simulink model "SMC"  (R2024b)
settings: Solver=FixedStepAuto  StartTime=0.0  StopTime=200  FixedStep=1e-3  RelTol=1e-3
undefined symbols (not defined in the file): Orientation, Position
libraries: robotlib x3, simulink_extras x3, sharedutil x2
(part 2 of 2)

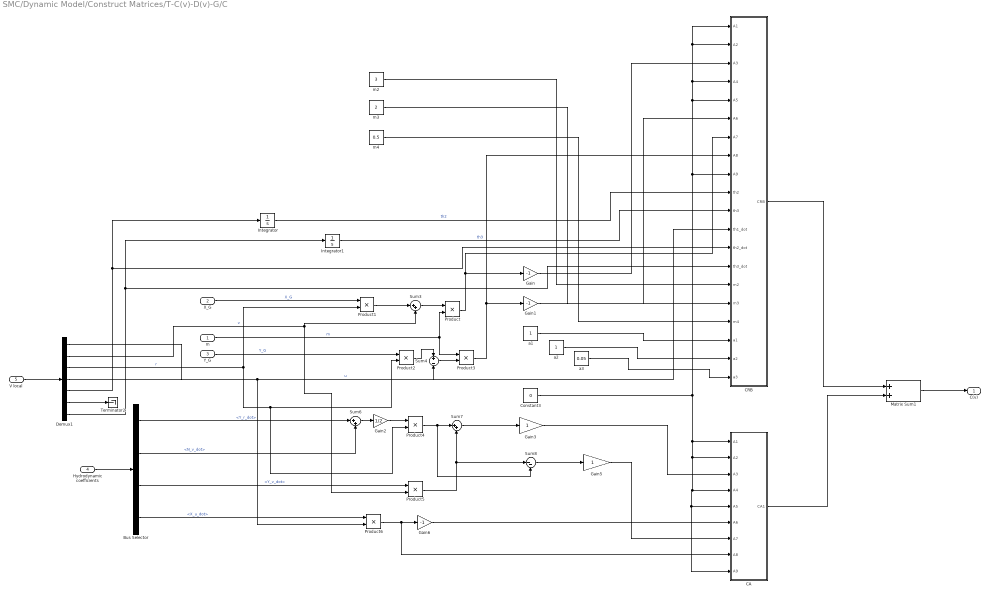
== system SMC/Dynamic Model/Construct Matrices/T-C(v)-D(v)-G/C ==
  m : Inport
  X_G : Inport  Port=2
  Y_G : Inport  Port=3
  Hydrodynamic coefficients : Inport  Port=4
  V local : Inport  Port=5
  Bus Selector : BusSelector  OutputSignals=Y_r_dot,N_v_dot,Y_v_dot,X_u_dot
  CA : MATLAB Function  TreatAsAtomicUnit=on
  CRB : MATLAB Function  TreatAsAtomicUnit=on
  Constant3 : Constant  Value=0
  Demux1 : Demux  Outputs=7
  Gain : Gain  Gain=-1
  Gain1 : Gain  Gain=-1
  Gain2 : Gain  Gain=1/2
  Gain3 : Gain
  Gain5 : Gain
  Gain6 : Gain  Gain=-1
  Integrator : Integrator
  Integrator1 : Integrator
  Matrix Sum1 : Sum
  Product{,1..6} (7 alike) : Product
  Sum3 : Sum  Inputs=|++
  Sum4 : Sum  Inputs=+-
  Sum6 : Sum  Inputs=|++
  Sum7 : Sum  Inputs=|++
  Sum8 : Sum  Inputs=|--
  Terminator2 : Terminator
  a1 : Constant
  a2 : Constant
  a3 : Constant  Value=0.05
  m2 : Constant  Value=3
  m3 : Constant  Value=2
  m4 : Constant  Value=0.5
  C(v) : Outport
  wires:
  Hydrodynamic coefficients/1 -> Bus Selector/1
  Demux1/1 -> Product6/2, Sum4/2  "u"
  Gain3/1 -> CA/3(A3)
  CRB/1(CRB) -> Matrix Sum1/1
  Demux1/4 -> CRB/12(th1_dot)
  Product1/1 -> Sum3/1
  Gain6/1 -> CA/6(A6)
  Constant3/1 -> CRB/9(A9), CRB/2(A2), CRB/1(A1), CRB/4(A4), CRB/5(A5), CA/4(A4), CA/5(A5), CA/9(A9), CA/2(A2), CA/1(A1)
  Bus Selector/1 -> Sum6/1  "<Y_r_dot>"
  Product6/1 -> Gain6/1, CA/8(A8)
  Y_G/1 -> Product2/1  "Y_G"
  Sum3/1 -> Product/1
  Demux1/2 -> Product5/2, Sum3/2  "v"
  Bus Selector/2 -> Sum6/2  "<N_v_dot>"
  Demux1/7 -> Integrator1/1, CRB/14(th3_dot)
  Gain1/1 -> CRB/6(A6)
  Sum6/1 -> Gain2/1
  X_G/1 -> Product1/1  "X_G"
  Product5/1 -> Sum7/2, Sum8/1
  Demux1/6 -> Terminator2/1
  Gain2/1 -> Product4/1
  Bus Selector/4 -> Product6/1  "<X_u_dot>"
  Product3/1 -> Gain1/1, CRB/8(A8)
  m/1 -> Product/2, Product3/1  "m"
  Gain/1 -> CRB/3(A3)
  Demux1/5 -> CRB/13(th2_dot), Integrator/1
  Product/1 -> Gain/1, CRB/7(A7)
  Product2/1 -> Sum4/1
  Demux1/3 -> Product1/2, Product2/2, Product4/2  "r"
  Sum7/1 -> Gain3/1
  Sum8/1 -> Gain5/1
  Bus Selector/3 -> Product5/1  "<Y_v_dot>"
  CA/1(CA1) -> Matrix Sum1/2
  Matrix Sum1/1 -> C(v)/1
  Gain5/1 -> CA/7(A7)
  Sum4/1 -> Product3/2
  V local/1 -> Demux1/1
  Product4/1 -> Sum7/1, Sum8/2
  Integrator/1 -> CRB/10(th2)  "th2"
  Integrator1/1 -> CRB/11(th3)  "th3"
  m2/1 -> CRB/15(m2)
  m3/1 -> CRB/16(m3)
  m4/1 -> CRB/17(m4)
  a1/1 -> CRB/18(a1)
  a2/1 -> CRB/19(a2)
  a3/1 -> CRB/20(a3)

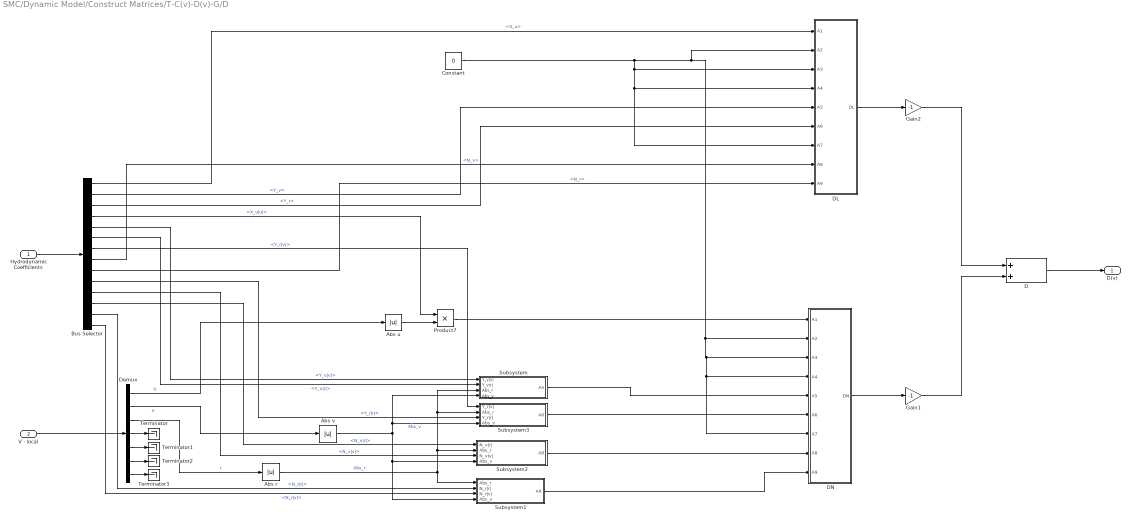
== system SMC/Dynamic Model/Construct Matrices/T-C(v)-D(v)-G/D ==
  note: u
  note: v
  Hydrodynamic Coefficients : Inport
  V - local : Inport  Port=2
  Abs r : Abs  SaturateOnIntegerOverflow=off
  Abs u : Abs  SaturateOnIntegerOverflow=off
  Abs v : Abs  SaturateOnIntegerOverflow=off
  Bus Selector : BusSelector  OutputSignals=X_u,Y_v,Y_r,X_u|u|,Y_v|v|,Y_v|r|,Y_r|v|,N_v,N_r,Y_r|r|,N_v|v|,N_v|r|,N_r|r|,N_r|v|
  Constant : Constant  Value=0
  D : Sum
  DL : MATLAB Function  TreatAsAtomicUnit=on
  DN : MATLAB Function  TreatAsAtomicUnit=on
  Demux : Demux  Outputs=7
  Gain1 : Gain  Gain=-1
  Gain2 : Gain  Gain=-1
  Product7 : Product
  Subsystem : Subsystem
  Subsystem1 : Subsystem
  Subsystem2 : Subsystem
  Subsystem3 : Subsystem
  Terminator{,1..3} (4 alike) : Terminator
  D(v) : Outport
  wires:
  Demux/7 -> Terminator3/1
  Hydrodynamic Coefficients/1 -> Bus Selector/1
  Demux/6 -> Terminator2/1
  Demux/5 -> Terminator1/1
  Demux/1 -> Abs u/1
  Demux/4 -> Terminator/1
  Bus Selector/5 -> Subsystem/1("Y_v|v| ")  "<Y_v|v|>"
  Demux/2 -> Abs v/1
  Abs r/1 -> Subsystem/3(Abs_r), Subsystem3/2("Abs_r "), Subsystem2/2(Abs_r), Subsystem1/1(Abs_r)  "Abs_r"
  Gain1/1 -> D/2
  DL/1(DL) -> Gain2/1
  DN/1(DN) -> Gain1/1
  V - local/1 -> Demux/1
  Bus Selector/6 -> Subsystem/2(Y_v|r|)  "<Y_v|r|>"
  Demux/3 -> Abs r/1  "r"
  D/1 -> D(v)/1
  Gain2/1 -> D/1
  Subsystem2/1(A8) -> DN/8(A8)
  Bus Selector/4 -> Product7/1  "<X_u|u|>"
  Bus Selector/13 -> Subsystem1/2(N_r|r|)  "<N_r|r|>"
  Bus Selector/11 -> Subsystem2/3(N_v|v|)  "<N_v|v|>"
  Bus Selector/12 -> Subsystem2/1(N_v|r|)  "<N_v|r|>"
  Subsystem1/1(A9) -> DN/9(A9)
  Bus Selector/7 -> Subsystem3/1(Y_r|v|)  "<Y_r|v|>"
  Abs v/1 -> Subsystem/4("Abs_v "), Subsystem3/4(Abs_v), Subsystem1/4(Abs_v), Subsystem2/4(Abs_v)  "Abs_v"
  Constant/1 -> DL/2(A2), DN/2(A2), DN/3(A3), DN/4(A4), DN/7(A7), DL/4(A4), DL/7(A7), DL/3(A3)
  Bus Selector/14 -> Subsystem1/3(N_r|v|)  "<N_r|v|>"
  Abs u/1 -> Product7/2
  Subsystem/1(A5) -> DN/5(A5)
  Bus Selector/1 -> DL/1(A1)  "<X_u>"
  Subsystem3/1(A6) -> DN/6(A6)
  Product7/1 -> DN/1(A1)
  Bus Selector/10 -> Subsystem3/3(Y_r|r|)  "<Y_r|r|>"
  Bus Selector/9 -> DL/9(A9)  "<N_r>"
  Bus Selector/8 -> DL/8(A8)  "<N_v>"
  Bus Selector/3 -> DL/6(A6)  "<Y_r>"
  Bus Selector/2 -> DL/5(A5)  "<Y_v>"

== system SMC/Dynamic Model/Construct Matrices/T-C(v)-D(v)-G/Tau ==
  B : Inport
  Tport : Inport  Port=2
  Tstbd : Inport  Port=3
  q1 : Inport  Port=4
  q2 : Inport  Port=5
  q3 : Inport  Port=6
  q4 : Inport  Port=7
  Mux : Mux  Inputs=7
  Product25 : Product
  Sum : Sum  Inputs=|++
  Sum1 : Sum  Inputs=|+-
  Ty : Constant  Value=0
  Tz : Gain  Gain=1/2
  T : Outport  VectorParamsAs1DForOutWhenUnconnected=off
  wires:
  Tstbd/1 -> Sum/2, Sum1/2  "Tstbd"
  q3/1 -> Mux/6
  q2/1 -> Mux/5
  q1/1 -> Mux/4
  Tz/1 -> Mux/3  "Tz"
  Product25/1 -> Tz/1
  Sum1/1 -> Product25/2
  Mux/1 -> T/1  "T"
  Tport/1 -> Sum/1, Sum1/1  "Tport"
  Ty/1 -> Mux/2  "Ty"
  Sum/1 -> Mux/1
  q4/1 -> Mux/7
  B/1 -> Product25/1  "B"

== system SMC/Controller/Construct Matrices/C(v)D(v)G/D/Subsystem ==
  "Y_v|v| " : Inport
  Y_v|r| : Inport  Port=2
  Abs_r : Inport  Port=3
  "Abs_v " : Inport  Port=4
  Product8 : Product
  Product9 : Product
  Sum10 : Sum  Inputs=|++
  A5 : Outport  VectorParamsAs1DForOutWhenUnconnected=off
  wires:
  Y_v|r|/1 -> Product9/1
  Abs_r/1 -> Product9/2
  Product9/1 -> Sum10/2
  "Y_v|v| "/1 -> Product8/1
  Product8/1 -> Sum10/1
  "Abs_v "/1 -> Product8/2
  Sum10/1 -> A5/1

== system SMC/Controller/Construct Matrices/C(v)D(v)G/D/Subsystem1 ==
  Abs_r : Inport
  N_r|r| : Inport  Port=2
  N_r|v| : Inport  Port=3
  Abs_v : Inport  Port=4
  Product14 : Product
  Product15 : Product
  Sum13 : Sum  Inputs=|++
  A9 : Outport  VectorParamsAs1DForOutWhenUnconnected=off
  wires:
  Product15/1 -> Sum13/1
  Sum13/1 -> A9/1
  N_r|v|/1 -> Product14/1
  Product14/1 -> Sum13/2
  Abs_r/1 -> Product15/2
  N_r|r|/1 -> Product15/1
  Abs_v/1 -> Product14/2

== system SMC/Controller/Construct Matrices/C(v)D(v)G/D/Subsystem2 ==
  N_v|r| : Inport
  Abs_r : Inport  Port=2
  N_v|v| : Inport  Port=3
  Abs_v : Inport  Port=4
  Product12 : Product
  Product13 : Product
  Sum12 : Sum  Inputs=|++
  A8 : Outport  VectorParamsAs1DForOutWhenUnconnected=off
  wires:
  Sum12/1 -> A8/1
  Product13/1 -> Sum12/1
  N_v|v|/1 -> Product12/1
  Product12/1 -> Sum12/2
  Abs_r/1 -> Product13/2
  Abs_v/1 -> Product12/2
  N_v|r|/1 -> Product13/1

== system SMC/Controller/Construct Matrices/C(v)D(v)G/D/Subsystem3 ==
  Y_r|v| : Inport
  "Abs_r " : Inport  Port=2
  Y_r|r| : Inport  Port=3
  Abs_v : Inport  Port=4
  Product10 : Product
  Product11 : Product
  Sum11 : Sum  Inputs=|++
  A6 : Outport  VectorParamsAs1DForOutWhenUnconnected=off
  wires:
  Product11/1 -> Sum11/2
  Product10/1 -> Sum11/1
  Sum11/1 -> A6/1
  Y_r|v|/1 -> Product10/1
  "Abs_r "/1 -> Product11/2
  Y_r|r|/1 -> Product11/1
  Abs_v/1 -> Product10/2

== system SMC/Dynamic Model/Construct Matrices/T-C(v)-D(v)-G/D/Subsystem ==
  "Y_v|v| " : Inport
  Y_v|r| : Inport  Port=2
  Abs_r : Inport  Port=3
  "Abs_v " : Inport  Port=4
  Product8 : Product
  Product9 : Product
  Sum10 : Sum  Inputs=|++
  A5 : Outport  VectorParamsAs1DForOutWhenUnconnected=off
  wires:
  Y_v|r|/1 -> Product9/1
  Abs_r/1 -> Product9/2
  Product9/1 -> Sum10/2
  "Y_v|v| "/1 -> Product8/1
  Product8/1 -> Sum10/1
  "Abs_v "/1 -> Product8/2
  Sum10/1 -> A5/1

== system SMC/Dynamic Model/Construct Matrices/T-C(v)-D(v)-G/D/Subsystem1 ==
  Abs_r : Inport
  N_r|r| : Inport  Port=2
  N_r|v| : Inport  Port=3
  Abs_v : Inport  Port=4
  Product14 : Product
  Product15 : Product
  Sum13 : Sum  Inputs=|++
  A9 : Outport  VectorParamsAs1DForOutWhenUnconnected=off
  wires:
  Product15/1 -> Sum13/1
  Sum13/1 -> A9/1
  N_r|v|/1 -> Product14/1
  Product14/1 -> Sum13/2
  Abs_r/1 -> Product15/2
  N_r|r|/1 -> Product15/1
  Abs_v/1 -> Product14/2

== system SMC/Dynamic Model/Construct Matrices/T-C(v)-D(v)-G/D/Subsystem2 ==
  N_v|r| : Inport
  Abs_r : Inport  Port=2
  N_v|v| : Inport  Port=3
  Abs_v : Inport  Port=4
  Product12 : Product
  Product13 : Product
  Sum12 : Sum  Inputs=|++
  A8 : Outport  VectorParamsAs1DForOutWhenUnconnected=off
  wires:
  Sum12/1 -> A8/1
  Product13/1 -> Sum12/1
  N_v|v|/1 -> Product12/1
  Product12/1 -> Sum12/2
  Abs_r/1 -> Product13/2
  Abs_v/1 -> Product12/2
  N_v|r|/1 -> Product13/1

== system SMC/Dynamic Model/Construct Matrices/T-C(v)-D(v)-G/D/Subsystem3 ==
  Y_r|v| : Inport
  "Abs_r " : Inport  Port=2
  Y_r|r| : Inport  Port=3
  Abs_v : Inport  Port=4
  Product10 : Product
  Product11 : Product
  Sum11 : Sum  Inputs=|++
  A6 : Outport  VectorParamsAs1DForOutWhenUnconnected=off
  wires:
  Product11/1 -> Sum11/2
  Product10/1 -> Sum11/1
  Sum11/1 -> A6/1
  Y_r|v|/1 -> Product10/1
  "Abs_r "/1 -> Product11/2
  Y_r|r|/1 -> Product11/1
  Abs_v/1 -> Product10/2

== matlab function SMC/MATLAB Function4 ==
  data: qw input; XYZ output; qx input; qy input; qz input
function XYZ = fcn(qw, qx, qy, qz)
quat = [qw qx qy qz];
XYZ = quat2eul(quat);

== matlab function SMC/Wave Disturbance ==
  data: t input; tau_wave output
function tau_wave = WaveDisturbance3DOF(t)
%#codegen
% Simulink-compatible wave disturbance force/torque for 3DOF USV

% Constants
rho = 1000;      % Water density [kg/m^3]
g = 9.81;        % Gravity [m/s^2]
L = 4.29;        % Length overall [m]
B = 2.20;        % Beam [m]
T = 0.105;       % Draft [m]
x_G = 1.27;      % CG longitudinal [m]

% Wave heading (0 = surge, pi/2 = sway)
beta = pi/4;     % 45 degrees in radians

% Wave properties (3 harmonic components)
A = [0.03, 0.04, 0.02];                % Amplitudes [m]
lambda = [2.0, 3.0, 1.5];             % Wavelengths [m]
omega = sqrt(g * 2 * pi ./ lambda);   % Angular frequencies [rad/s]
phi = [0, pi/4, pi/2];                % Phases

% Initialize slope s_i(t)
s = zeros(1,3);
for i = 1:3
    s(i) = (A(i)/(2*pi*lambda(i))) * sin(omega(i)*t + phi(i));
end

% Compute wave-induced forces
X_wave = sum(rho * g * B * L * T * cos(beta) * s);
Y_wave = -sum(rho * g * B * L * T * sin(beta) * s);
N_wave = sum((1/24) * rho * g * B * L * (L^2 - B^2) * sin(2*beta) * s.^2);

% Output vector
tau_wave = [X_wave; Y_wave; N_wave; 0; 0; 0; 0];

== matlab function SMC/Controller/Subsystem5/MATLAB Function ==
  data: A1 input; A2 input; A3 input; A4 input; A5 input; A6 input; A7 input; A8 input; A9 input; J1 output
function J1 = fcn(A1, A2, A3, A4, A5, A6, A7, A8, A9)

J1 = [A1,A2,A3,0,0,0,0;
    A4,A5,A6,0,0,0,0;
    A7,A8,A9,0,0,0,0;
    0,0,0,1,0,0,0;
    0,0,0,0,1,0,0;
    0,0,0,0,0,1,0;
    0,0,0,0,0,0,1;];

== matlab function SMC/Dynamic Model/Construct Matrices/M/MATLAB Function ==
  data: A1 input; A2 input; A3 input; A4 input; A5 input; A6 input; A7 input; A8 input; A9 input; M output; m1 input; m2 input; m3 input; m4 input; a1 input; a2 input; a3 input; th2 input; th3 input
function M = fcn(A1, A2, A3, A4, A5, A6, A7, A8, A9, m1, m2, m3, m4, a1, a2, a3, th2, th3)

% Define the expressions for M
m11 = (a1^2*m1)/4 + a1^2*m2 + a1^2*m3 + (a2^2*m2)/4 + a1^2*m4 + a2^2*m3 + a2^2*m4 + a3^2*m4 + 2*a1*a3*m4*cos(th2 + th3) + a1*a2*m2*cos(th2) + 2*a1*a2*m3*cos(th2) + 2*a1*a2*m4*cos(th2) + 2*a2*a3*m4*cos(th3);
m12 = (a2^2*m2)/4 + a2^2*m3 + a2^2*m4 + a3^2*m4 + a1*a3*m4*cos(th2 + th3) + (a1*a2*m2*cos(th2))/2 + a1*a2*m3*cos(th2) + a1*a2*m4*cos(th2) + 2*a2*a3*m4*cos(th3);
m13 = 0;
m14 = a3^2*m4 + a1*a3*m4*cos(th2 + th3) + a2*a3*m4*cos(th3);
m21 = (a2^2*m2)/4 + a2^2*m3 + a2^2*m4 + a3^2*m4 + a1*a3*m4*cos(th2 + th3) + (a1*a2*m2*cos(th2))/2 + a1*a2*m3*cos(th2) + a1*a2*m4*cos(th2) + 2*a2*a3*m4*cos(th3);
m22 = (a2^2*m2)/4 + a2^2*m3 + a2^2*m4 + a3^2*m4 + 2*a2*a3*m4*cos(th3);
m23 = 0;
m24 = m4*a3^2 + a2*m4*cos(th3)*a3;
m31 = 0;
m32 = 0;
m33 = (m3 + 4*m4)/4;
m34 = 0;
m41 = a3^2*m4 + a3*m4*a1*cos(th2 + th3) + a3*m4*a2*cos(th3);
m42 = a3^2*m4 + a3*m4*a2*cos(th3);
m43 = 0;
m44 = a3^2*m4;

M = [A1,A2,A3,0,0,0,0;
    A4,A5,A6,0,0,0,0;
    A7,A8,A9,0,0,0,0;
    0,0,0,m11,m12,m13,m14;
    0,0,0,m21,m22,m23,m24;
    0,0,0,m31,m32,m33,m34;
    0,0,0,m41,m42,m43,m44];

== matlab function SMC/Dynamic Model/Construct Matrices/M^-1 ==
  data: u input; y output
function y = fcn(u)
y = inv(u);

== matlab function SMC/Dynamic Model/Construct Matrices/T-C(v)-D(v)-G/C/CA ==
  data: A1 input; A2 input; A3 input; A4 input; A5 input; A6 input; A7 input; A8 input; A9 input; CA1 output
function CA1 = fcn(A1, A2, A3, A4, A5, A6, A7, A8, A9)

CA1 = [A1,A2,A3,0,0,0,0;
    A4,A5,A6,0,0,0,0;
    A7,A8,A9,0,0,0,0;
    0,0,0,0,0,0,0;
    0,0,0,0,0,0,0;
    0,0,0,0,0,0,0;
    0,0,0,0,0,0,0;];

== matlab function SMC/Dynamic Model/Construct Matrices/T-C(v)-D(v)-G/C/CRB ==
  data: A1 input; A2 input; A3 input; A4 input; A5 input; A6 input; A7 input; A8 input; A9 input; CRB output; th2 input; th3 input; th1_dot input; th2_dot input; th3_dot input; m2 input; m3 input; m4 input; a1 input; a2 input; a3 input
function CRB = fcn(A1, A2, A3, A4, A5, A6, A7, A8, A9, th2, th3, th1_dot, th2_dot, th3_dot, m2, m3, m4, a1, a2, a3)

% Define the expressions for C
c11 = -2*a1*a3*m4*sin(th2 + th3) + th2_dot + th3_dot - a1*a2*m2*sin(th2) - 2*a1*a2*m3*sin(th2) - 2*a1*a2*m4*sin(th2) - 2*a2*a3*m4*sin(th3);
c12 = -a1*a3*m4*sin(th2 + th3) + th2_dot + th3_dot - (a1*a2*m2*sin(th2))/2 - a1*a2*m3*sin(th2) - a1*a2*m4*sin(th2) - 2*a2*a3*m4*sin(th3);
c13 = 0;
c14 = -a1*a3*m4*sin(th2 + th3) + th2_dot + th3_dot - a2*a3*m4*sin(th3);
c21 = ((a1*(a2*m2*sin(th2) + 2*a2*m3*sin(th2) + 2*a2*m4*sin(th2) + 2*a3*m4*sin(th2 + th3)))/2)*th1_dot + - a1*a3*m4*sin(th2 + th3) - (a1*a2*m2*sin(th2))/2 - a1*a2*m3*sin(th2) - a1*a2*m4*sin(th2) - 2*a2*a3*m4*sin(th3);
c22 = ((a1*(a2*m2*sin(th2) + 2*a2*m3*sin(th2) + 2*a2*m4*sin(th2) + 2*a3*m4*sin(th2 + th3)))/2 + 1)*th1_dot - 2*a2*a3*m4*sin(th3);
c23 = 0;
c24 = (a1*a3*m4*sin(th2 + th3) + 1)*th1_dot - a2*a3*m4*sin(th3);
c31 = 0;
c32 = 0;
c33 = 0;
c34 = 0;
c41 = a2*sin(th3)*th1_dot - a1*a3*m4*sin(th2 + th3) - a2*a3*m4*sin(th3);
c42 = (a3*m4*(a1*sin(th2 + th3) + a2*sin(th3)) + a2*a3*m4*sin(th3) + 1)*th1_dot + a2*a3*m4*sin(th3)*th2_dot -a2*a3*m4*sin(th3);
c43 = 0;
c44 = a2*a3*m4*sin(th3)*th2_dot + (a3*m4*(a1*sin(th2 + th3) + a2*sin(th3)) + 1)*th1_dot;

CRB = [A1,A2,A3,0,0,0,0;
    A4,A5,A6,0,0,0,0;
    A7,A8,A9,0,0,0,0;
    0,0,0,c11,c12,c13,c14;
    0,0,0,c21,c22,c23,c24;
    0,0,0,c31,c32,c33,c34;
    0,0,0,c41,c42,c43,c44];

== matlab function SMC/Dynamic Model/Construct Matrices/T-C(v)-D(v)-G/D/DL ==
  data: A1 input; A2 input; A3 input; A4 input; A5 input; A6 input; A7 input; A8 input; A9 input; DL output
function DL = fcn(A1, A2, A3, A4, A5, A6, A7, A8, A9)

DL = [A1,A2,A3,0,0,0,0;
    A4,A5,A6,0,0,0,0;
    A7,A8,A9,0,0,0,0;
    0,0,0,0,0,0,0;
    0,0,0,0,0,0,0;
    0,0,0,0,0,0,0;
    0,0,0,0,0,0,0;];

== matlab function SMC/Dynamic Model/Construct Matrices/T-C(v)-D(v)-G/D/DN ==
  data: A1 input; A2 input; A3 input; A4 input; A5 input; A6 input; A7 input; A8 input; A9 input; DN output
function DN = fcn(A1, A2, A3, A4, A5, A6, A7, A8, A9)

DN = [A1,A2,A3,0,0,0,0;
    A4,A5,A6,0,0,0,0;
    A7,A8,A9,0,0,0,0;
    0,0,0,0,0,0,0;
    0,0,0,0,0,0,0;
    0,0,0,0,0,0,0;
    0,0,0,0,0,0,0];

== matlab function SMC/Dynamic Model/Construct Matrices/T-C(v)-D(v)-G/G ==
  data: m3 input; G output; m4 input; g input
function G = fcn(m3, m4, g)

% Define the expressions for G
g1 = 0
g2 = 0
g3 = g*(m3 + m4)
g4 = 0

G = [0;0;0;g1;g2;g3;g4];

== matlab function SMC/Controller/Construct Matrices/M2/MATLAB Function ==
  data: A1 input; A2 input; A3 input; A4 input; A5 input; A6 input; A7 input; A8 input; A9 input; M output; m1 input; m2 input; m3 input; m4 input; a1 input; a2 input; a3 input; th2 input; th3 input
function M = fcn(A1, A2, A3, A4, A5, A6, A7, A8, A9, m1, m2, m3, m4, a1, a2, a3, th2, th3)

% Define the expressions for M
m11 = (a1^2*m1)/4 + a1^2*m2 + a1^2*m3 + (a2^2*m2)/4 + a1^2*m4 + a2^2*m3 + a2^2*m4 + a3^2*m4 + 2*a1*a3*m4*cos(th2 + th3) + a1*a2*m2*cos(th2) + 2*a1*a2*m3*cos(th2) + 2*a1*a2*m4*cos(th2) + 2*a2*a3*m4*cos(th3);
m12 = (a2^2*m2)/4 + a2^2*m3 + a2^2*m4 + a3^2*m4 + a1*a3*m4*cos(th2 + th3) + (a1*a2*m2*cos(th2))/2 + a1*a2*m3*cos(th2) + a1*a2*m4*cos(th2) + 2*a2*a3*m4*cos(th3);
m13 = 0;
m14 = a3^2*m4 + a1*a3*m4*cos(th2 + th3) + a2*a3*m4*cos(th3);
m21 = (a2^2*m2)/4 + a2^2*m3 + a2^2*m4 + a3^2*m4 + a1*a3*m4*cos(th2 + th3) + (a1*a2*m2*cos(th2))/2 + a1*a2*m3*cos(th2) + a1*a2*m4*cos(th2) + 2*a2*a3*m4*cos(th3);
m22 = (a2^2*m2)/4 + a2^2*m3 + a2^2*m4 + a3^2*m4 + 2*a2*a3*m4*cos(th3);
m23 = 0;
m24 = m4*a3^2 + a2*m4*cos(th3)*a3;
m31 = 0;
m32 = 0;
m33 = (m3 + 4*m4)/4;
m34 = 0;
m41 = a3^2*m4 + a3*m4*a1*cos(th2 + th3) + a3*m4*a2*cos(th3);
m42 = a3^2*m4 + a3*m4*a2*cos(th3);
m43 = 0;
m44 = a3^2*m4;

M = [A1,A2,A3,0,0,0,0;
    A4,A5,A6,0,0,0,0;
    A7,A8,A9,0,0,0,0;
    0,0,0,m11,m12,m13,m14;
    0,0,0,m21,m22,m23,m24;
    0,0,0,m31,m32,m33,m34;
    0,0,0,m41,m42,m43,m44];

== matlab function SMC/Controller/Construct Matrices/C(v)D(v)G/C/CA ==
  data: A1 input; A2 input; A3 input; A4 input; A5 input; A6 input; A7 input; A8 input; A9 input; CA1 output
function CA1 = fcn(A1, A2, A3, A4, A5, A6, A7, A8, A9)

CA1 = [A1,A2,A3,0,0,0,0;
    A4,A5,A6,0,0,0,0;
    A7,A8,A9,0,0,0,0;
    0,0,0,0,0,0,0;
    0,0,0,0,0,0,0;
    0,0,0,0,0,0,0;
    0,0,0,0,0,0,0;];

== matlab function SMC/Controller/Construct Matrices/C(v)D(v)G/C/CRB ==
  data: A1 input; A2 input; A3 input; A4 input; A5 input; A6 input; A7 input; A8 input; A9 input; CRB output; th2 input; th3 input; th1_dot input; th2_dot input; th3_dot input; m2 input; m3 input; m4 input; a1 input; a2 input; a3 input
function CRB = fcn(A1, A2, A3, A4, A5, A6, A7, A8, A9, th2, th3, th1_dot, th2_dot, th3_dot, m2, m3, m4, a1, a2, a3)

% Define the expressions for C
c11 = -2*a1*a3*m4*sin(th2 + th3) + th2_dot + th3_dot - a1*a2*m2*sin(th2) - 2*a1*a2*m3*sin(th2) - 2*a1*a2*m4*sin(th2) - 2*a2*a3*m4*sin(th3);
c12 = -a1*a3*m4*sin(th2 + th3) + th2_dot + th3_dot - (a1*a2*m2*sin(th2))/2 - a1*a2*m3*sin(th2) - a1*a2*m4*sin(th2) - 2*a2*a3*m4*sin(th3);
c13 = 0;
c14 = -a1*a3*m4*sin(th2 + th3) + th2_dot + th3_dot - a2*a3*m4*sin(th3);
c21 = ((a1*(a2*m2*sin(th2) + 2*a2*m3*sin(th2) + 2*a2*m4*sin(th2) + 2*a3*m4*sin(th2 + th3)))/2)*th1_dot + - a1*a3*m4*sin(th2 + th3) - (a1*a2*m2*sin(th2))/2 - a1*a2*m3*sin(th2) - a1*a2*m4*sin(th2) - 2*a2*a3*m4*sin(th3);
c22 = ((a1*(a2*m2*sin(th2) + 2*a2*m3*sin(th2) + 2*a2*m4*sin(th2) + 2*a3*m4*sin(th2 + th3)))/2 + 1)*th1_dot - 2*a2*a3*m4*sin(th3);
c23 = 0;
c24 = (a1*a3*m4*sin(th2 + th3) + 1)*th1_dot - a2*a3*m4*sin(th3);
c31 = 0;
c32 = 0;
c33 = 0;
c34 = 0;
c41 = a2*sin(th3)*th1_dot - a1*a3*m4*sin(th2 + th3) - a2*a3*m4*sin(th3);
c42 = (a3*m4*(a1*sin(th2 + th3) + a2*sin(th3)) + a2*a3*m4*sin(th3) + 1)*th1_dot + a2*a3*m4*sin(th3)*th2_dot -a2*a3*m4*sin(th3);
c43 = 0;
c44 = a2*a3*m4*sin(th3)*th2_dot + (a3*m4*(a1*sin(th2 + th3) + a2*sin(th3)) + 1)*th1_dot;

CRB = [A1,A2,A3,0,0,0,0;
    A4,A5,A6,0,0,0,0;
    A7,A8,A9,0,0,0,0;
    0,0,0,c11,c12,c13,c14;
    0,0,0,c21,c22,c23,c24;
    0,0,0,c31,c32,c33,c34;
    0,0,0,c41,c42,c43,c44];

== matlab function SMC/Controller/Construct Matrices/C(v)D(v)G/D/DL ==
  data: A1 input; A2 input; A3 input; A4 input; A5 input; A6 input; A7 input; A8 input; A9 input; DL output
function DL = fcn(A1, A2, A3, A4, A5, A6, A7, A8, A9)

DL = [A1,A2,A3,0,0,0,0;
    A4,A5,A6,0,0,0,0;
    A7,A8,A9,0,0,0,0;
    0,0,0,0,0,0,0;
    0,0,0,0,0,0,0;
    0,0,0,0,0,0,0;
    0,0,0,0,0,0,0;];

== matlab function SMC/Controller/Construct Matrices/C(v)D(v)G/D/DN ==
  data: A1 input; A2 input; A3 input; A4 input; A5 input; A6 input; A7 input; A8 input; A9 input; DN output
function DN = fcn(A1, A2, A3, A4, A5, A6, A7, A8, A9)

DN = [A1,A2,A3,0,0,0,0;
    A4,A5,A6,0,0,0,0;
    A7,A8,A9,0,0,0,0;
    0,0,0,0,0,0,0;
    0,0,0,0,0,0,0;
    0,0,0,0,0,0,0;
    0,0,0,0,0,0,0;];

== matlab function SMC/Controller/Construct Matrices/C(v)D(v)G/G ==
  data: m3 input; G output; m4 input; g input
function G = fcn(m3, m4, g)

% Define the expressions for G
g1 = 0
g2 = 0
g3 = g*(m3 + m4)
g4 = 0

G = [0;0;0;g1;g2;g3;g4];

== matlab function SMC/MATLAB Function1 ==
  data: th1 input; T output; th2 input; d input; th3 input; h input; L1 input; L2 input; L3 input
function T = fcn(th1, th2, d,th3, h, L1, L2, L3)
T = [cos(th1 + th2 + th3), -sin(th1 + th2 + th3), 0, L1*cos(th1) + L2*cos(th1 + th2) + L3*cos(th1 + th2 + th3);
    sin(th1 + th2 + th3), cos(th1 + th2 + th3), 0, L1*sin(th1) + L2*sin(th1 + th2) + L3*sin(th1 + th2 + th3);
    0, 0, 1, h-d;
    0,0,0,1];

== matlab function SMC/Controller/MATLAB Function ==
  data: u input; y output
function y = fcn(u)

y = inv(u);

== matlab function SMC/MATLAB Function2 ==
  data: Px input; Py input; Pz input; L1 input; L2 input; h input; q1 output; q2 output; q3 output; q4 output
function [q1, q2, q3, q4] = fcn(Px,Py,Pz,L1,L2,h)

c2 = (Px^2 + Py^2 - L1^2 - L2^2)/(2*L1*L2);

q2 = acos((Px^2 + Py^2 - L1^2 - L2^2)/(2*L1*L2));
q1 = atan((-L2*sin(q2)*Px + (L1 + L2*cos(q2))*Py)/(L2*sin(q2)*Py + (L1 + L2*cos(q2))*Px));
q3 = Pz-h;
a = sin(q1 + q2);
b = cos(q1 + q2);
q4 = atan(-a/b)-q1-q2;
